simulink model "StateSpaceController"  (R2021a)
settings: Solver=FixedStepAuto  StartTime=0.0  StopTime=SimTime-Ts  FixedStep=1e-3  RelTol=1e-3
values from neighbouring files (symbols this model uses):
  b0 = B_q(1)    [PIDModalController.m]    (also in PolynomialController.m)
  C12 = x(3)    [DigitalPIDRunner.m]    (also in DoubleMassRunner.m; NNIdentify.m = Xnt_noise(3); NNTrainingSet.m = T(i, 3); PIDModalController.m = 16.6338)
  k1 = x(1)    [DigitalPIDRunner.m]    (also in DoubleMassRunner.m; NNIdentify.m = Xnt_noise(1); NNTrainingSet.m = T(i, 1); PIDModalController.m = 0.2244)
  k2 = x(2)    [DigitalPIDRunner.m]    (also in DoubleMassRunner.m; NNIdentify.m = Xnt_noise(2); NNTrainingSet.m = T(i, 2); PIDModalController.m = 0.5636)
  Ts = 1e-3    (= 0.001)    [DigitalPIDRunner.m]    (also in DoubleMassRunner.m = ref.Ts; NNTrainingSet.m; PIDModalController.m; PIDRunner.m = p.Results.StepTime)
undefined symbols (not defined in the file or in its folder): b1, dss0, K
settings Model: Creator=akangmufti  LastModifiedBy=akangmufti

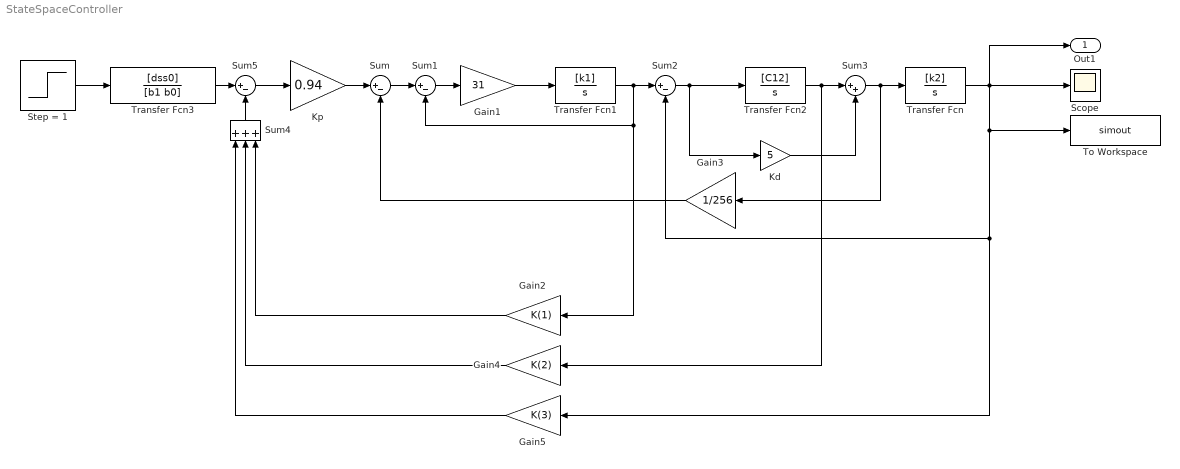
== system StateSpaceController ==
  Gain1 : Gain  Gain=31
  Gain2 : Gain  Gain=K(1)
  Gain3 : Gain  Gain=1/256
  Gain4 : Gain  Gain=K(2)
  Gain5 : Gain  Gain=K(3)
  Kd : Gain  Gain=5
  Kp : Gain  Gain=0.94
  Scope : Scope
  Step = 1 : Step  Time=0.0001  SampleTime=0
  Sum{,1..2,5} (4 alike) : Sum  Inputs=|+-
  Sum3 : Sum  Inputs=|++
  Sum4 : Sum  Inputs=+++
  To Workspace : ToWorkspace  VariableName=simout  SampleTime=Ts
      settings: Save2DSignal=2-D array (concatenate along first dimension)
  Transfer Fcn : TransferFcn  Numerator=[k2]  Denominator=[1 0]  ContinuousStateAttributes='x3'
  Transfer Fcn1 : TransferFcn  Numerator=[k1]  Denominator=[1 0]  ContinuousStateAttributes='x1'
  Transfer Fcn2 : TransferFcn  Numerator=[C12]  Denominator=[1 0]  ContinuousStateAttributes='x2'
  Transfer Fcn3 : TransferFcn  Numerator=[dss0]  Denominator=[b1 b0]  ContinuousStateAttributes='x1'
  Out1 : Outport
  wires:
  Transfer Fcn/1 -> Scope/1, Out1/1, Gain5/1, Sum2/2, To Workspace/1
  Kd/1 -> Sum3/2
  Transfer Fcn2/1 -> Gain4/1, Sum3/1
  Sum3/1 -> Gain3/1, Transfer Fcn/1
  Sum/1 -> Sum1/1
  Gain3/1 -> Sum/2
  Sum1/1 -> Gain1/1
  Sum2/1 -> Kd/1, Transfer Fcn2/1
  Gain1/1 -> Transfer Fcn1/1
  Transfer Fcn1/1 -> Gain2/1, Sum1/2, Sum2/1
  Kp/1 -> Sum/1
  Gain2/1 -> Sum4/3
  Gain4/1 -> Sum4/2
  Gain5/1 -> Sum4/1
  Sum4/1 -> Sum5/2
  Sum5/1 -> Kp/1
  Transfer Fcn3/1 -> Sum5/1
  Step = 1/1 -> Transfer Fcn3/1
